simulink model "sm_dump_trailer"  (R2021b)
settings: Solver=VariableStepAuto  StartTime=0.0  StopTime=10  FixedStep=0.0001  RelTol=1e-3  AbsTol=1e-3  EnableMultiTasking=on
model workspace: external: MATLAB File sm_dump_trailer_params.m (data not in the file)
undefined symbols (not defined in the file or in its folder): base, bed, cylinder, lowerarm, sigbuilder_block, upperarm, X, Y, Z
libraries: sm_lib x65, sm_dump_trailer_lib x20, fl_lib x7, nesl_utility x4, simulink x4, sm_interface_elements_lib x1
(part 1 of 3)
CloseFcn:
  | clear simlog_sm_dump_trailer
Description:
  | Hydraulic Interface - Dump Trailer with Hydraulic Cylinder
settings Model: Creator=The MathWorks, Inc.  LastModifiedBy=The MathWorks, Inc.
settings SolverCC: AutoScaleAbsTol=off  AlgebraicLoopSolver=TrustRegion
settings DataIOCC: SaveFormat=StructureWithTime  SaveOutput=off  SignalLogging=off  DSMLogging=off  SaveTime=off  ReturnWorkspaceOutputs=off  ReturnWorkspaceOutputsName=spidata
settings DebuggingCC: SFMachineParentedDataDiag=warning  ArithmeticOperatorsInVariantConditions=warning
settings SFSimCC: SimUseLocalCustomCode=off  CustomCodeUndefinedFunction=UseInterfaceOnly
settings RTWCC: RTWUseLocalCustomCode=off
settings CodeAppCC: StateflowObjectComments=on
settings GRTTargetCC: TargetLangStandard=C89/C90 (ANSI)
settings ConfigComp: CovMetricSettings=dw  CovSaveCumulativeToWorkspaceVar=on  CovSaveSingleToWorkspaceVar=on  CovExternalEMLEnable=off
settings SimscapeCC: SimscapeNormalizeSystem=off  SimscapeLogType=all  SimscapeLogSimulationStatistics=on  SimscapeLogName=simlog_sm_dump_trailer  SimscapeLogDataHistory=10000
settings ExplorerConfigSet: InternalSimMechanicsExplorerSettings="<ExplorerConfiguration><canonicalview>default</canonicalview><AnimationSetting><BasePlaybackSpeed>1.0</BasePlaybackSpeed><PlaybackSpeedFactor>1.0</PlaybackSpeedFactor></AnimationSetting><TilePanel><TileInfo><Tiles Columns=\"1\" Count=\"1\" Rows=\"1\"><Column Left=\"2\" Weight=\"1\"/><Column Left=\"535\"/><Row Top=\"2\" Weight=\"1\"/><Row Top=\"498\"/><Tile Height=\"1\" Width=\"1\" X=\"0\" Y=\"0\"/></Tiles></TileInfo><SceneInfo><SceneViewer><BGColor><R>0.60000002384185791</R><G>0.60000002384185791</G><B>0.60000002384185791</B></BGColor><Camera><DoPerspective>off</DoPerspective><Position><X>1.5277086158018158</X><Y>0.21029843104978743</Y><Z>2.2318283328195734</Z></Position><Center><X>-0.21869209269767445</X><Y>1.956699139549277</Y><Z>0.48542762432009623</Z></Center><Up><X>-0.40824829046386307</X><Y>0.40824829046386307</Y><Z>0.81649658092772615</Z></Up><ViewLimDist>1</ViewLimDist><YLim>1.9305354565325132</YLim><XLim>2.0772085815668109</XLim></Camera></SceneViewer></SceneInfo></TilePanel><MechEditorPanel><Cameras/><GfxPanelCameraMap/><VideoCreator><PlaybackSpeedRatio>1.0</PlaybackSpeedRatio><FrameRate>30</FrameRate><VideoFormat>Motion JPEG AVI</VideoFormat><FrameSize>auto</FrameSize></VideoCreator></MechEditorPanel></ExplorerConfiguration>"

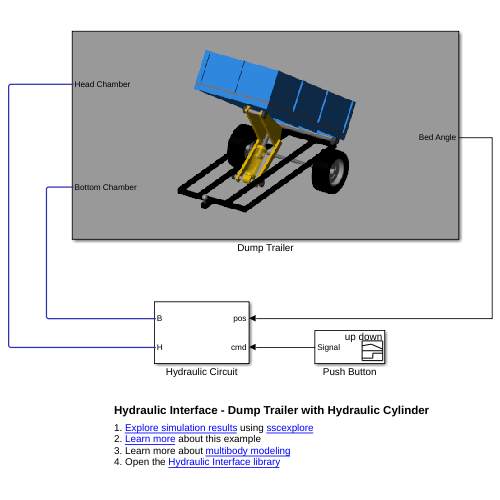
[thumbnail: Simulink's stored preview of the top-level diagram]
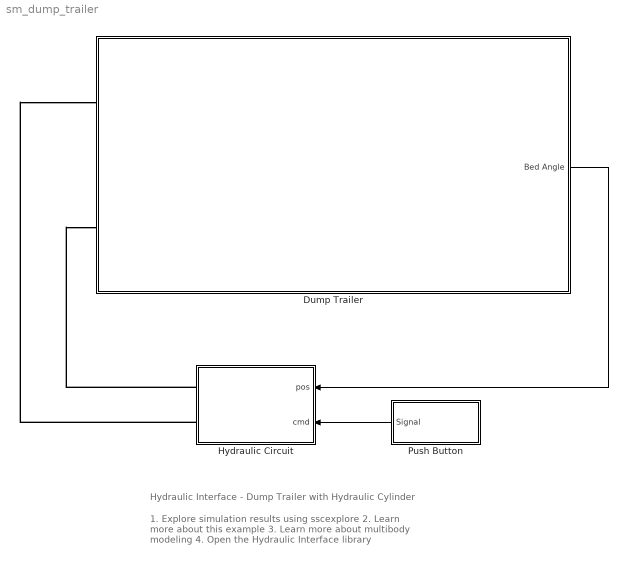
== system sm_dump_trailer ==
  note: Hydraulic Interface - Dump Trailer with Hydraulic Cylinder
  note: 1. Explore simulation results using sscexplore
      | 2. Learn more about this example
      | 3. Learn more about multibody modeling
      | 4. Open the Hydraulic Interface library
  Dump Trailer : Subsystem
      mask Display: image(fullfile(matlabroot,'toolbox','physmod','sm','smdemos','dump_trailer','images','sm_dump_trailer.png'));
  Hydraulic Circuit : Subsystem
  Push Button : Subsystem  Tag=STV Subsys  LoadFcn=sigbuilder_block('load');  StartFcn=sigbuilder_block('start');  StopFcn=sigbuilder_block('stop');  ClipboardFcn=sigbuilder_block('clipboard');  mask(Sigbuilder block){tuvar=[0:10]}
      mask help: Simulink:masks:SigbuilderBlock_MD
      mask init:
      | if ~strcmp(get_param(bdroot(gcbh),'SimulationStatus'),'stopped') tuvar = sigbuilder_block('maskInit'); end
      settings: CopyFcn=sigbuilder_block('copy');  DeleteFcn=sigbuilder_block('delete');  ModelCloseFcn=sigbuilder_block('modelClose');  PreSaveFcn=sigbuilder_block('preSave');  PauseFcn=sigbuilder_block('pause');  ContinueFcn=sigbuilder_block('continue');  NameChangeFcn=sigbuilder_block('namechange');  OpenFcn=sigbuilder_block('open',[547.5 174.75 550.5 399.75 ]);  CloseFcn=sigbuilder_block('close');
      mask Display: plot(0, 0, 100, 100,[2, 2, 32, 32, 2], [68, 8, 8, 68, 68],[32, 2], [38, 38], [32, 19, 2],[53, 60, 44], [32, 17, 17, 2],[16, 16, 31, 31]);txt = getActiveGroup(gcbh);text(2, 100, txt,'verticalAlignment', 'top');
  wires:
  Dump Trailer/1(Bed Angle) -> Hydraulic Circuit/2(pos)
  Push Button/1(Signal) -> Hydraulic Circuit/1(cmd)
  connections:
  Hydraulic Circuit/RConn2 -- Dump Trailer/LConn2
  Hydraulic Circuit/RConn1 -- Dump Trailer/LConn1

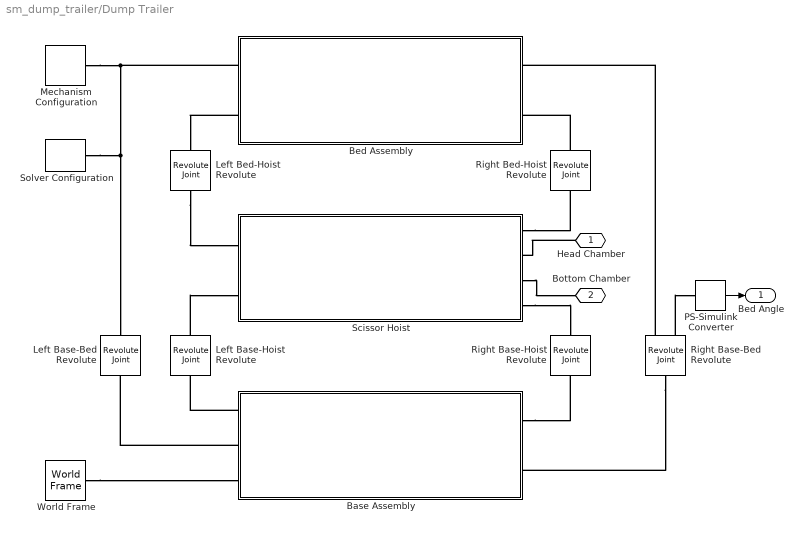
== system sm_dump_trailer/Dump Trailer ==
  Base Assembly : Subsystem
      mask Display: image(fullfile(matlabroot,'toolbox','physmod','sm','smdemos','dump_trailer','images','sm_dump_trailer_base_assembly.png'));
  Bed Assembly : Subsystem
      mask Display: image(fullfile(matlabroot,'toolbox','physmod','sm','smdemos','dump_trailer','images','sm_dump_trailer_bed_assembly.png'));
  Left Base-Bed Revolute : sm_lib/Joints/Revolute Joint  JointMode=Normal  SenseConstraintForce=off  SenseConstraintForceX=off  SenseConstraintForceY=off  SenseConstraintForceZ=off  SenseConstraintTorque=off  SenseConstraintTorqueX=off  SenseConstraintTorqueY=off  SenseConstraintTorqueZ=off  SenseTotalForce=off  SenseTotalForceX=off  SenseTotalForceY=off  SenseTotalForceZ=off  SenseTotalTorque=off  SenseTotalTorqueX=off  SenseTotalTorqueY=off  SenseTotalTorqueZ=off  CompositeWrenchDir=FollowerOnBase  CompositeWrenchFrame=BaseFrame  EquilibriumPosition=0  EquilibriumPositionUnits=deg  SpringStiffness=0  SpringStiffnessUnits=N*m/deg  DampingCoefficient=0  DampingCoefficientUnits=N*m/(deg/s)  TorqueActuationMode=NoTorque  MotionActuationMode=ComputedMotion  SensePosition=off  SenseVelocity=off  SenseAcceleration=off  SenseTorqueForce=off  SenseLowerLimitTorqueForce=off  SenseUpperLimitTorqueForce=off  LowerLimitSpecify=off  LowerLimitBound=-90  LowerLimitBoundUnits=deg  LowerLimitStiffness=1e4  LowerLimitStiffnessUnits=N*m/deg  LowerLimitDamping=10  LowerLimitDampingUnits=N*m/(deg/s)  LowerLimitTransitionRegionWidth=0.1  LowerLimitTransitionRegionWidthUnits=deg  UpperLimitSpecify=off  UpperLimitBound=90  UpperLimitBoundUnits=deg  UpperLimitStiffness=1e4  UpperLimitStiffnessUnits=N*m/deg  UpperLimitDamping=10  UpperLimitDampingUnits=N*m/(deg/s)  UpperLimitTransitionRegionWidth=0.1  UpperLimitTransitionRegionWidthUnits=deg  PositionTargetSpecify=off  PositionTargetPriority=High  PositionTargetValue=180  PositionTargetValueUnits=deg  VelocityTargetSpecify=off  VelocityTargetPriority=High  VelocityTargetValue=0  VelocityTargetValueUnits=deg/s
  Left Base-Hoist Revolute : sm_lib/Joints/Revolute Joint  JointMode=Normal  SenseConstraintForce=off  SenseConstraintForceX=off  SenseConstraintForceY=off  SenseConstraintForceZ=off  SenseConstraintTorque=off  SenseConstraintTorqueX=off  SenseConstraintTorqueY=off  SenseConstraintTorqueZ=off  SenseTotalForce=off  SenseTotalForceX=off  SenseTotalForceY=off  SenseTotalForceZ=off  SenseTotalTorque=off  SenseTotalTorqueX=off  SenseTotalTorqueY=off  SenseTotalTorqueZ=off  CompositeWrenchDir=FollowerOnBase  CompositeWrenchFrame=BaseFrame  EquilibriumPosition=0  EquilibriumPositionUnits=deg  SpringStiffness=0  SpringStiffnessUnits=N*m/deg  DampingCoefficient=0  DampingCoefficientUnits=N*m/(deg/s)  TorqueActuationMode=NoTorque  MotionActuationMode=ComputedMotion  SensePosition=off  SenseVelocity=off  SenseAcceleration=off  SenseTorqueForce=off  SenseLowerLimitTorqueForce=off  SenseUpperLimitTorqueForce=off  LowerLimitSpecify=off  LowerLimitBound=-90  LowerLimitBoundUnits=deg  LowerLimitStiffness=1e4  LowerLimitStiffnessUnits=N*m/deg  LowerLimitDamping=10  LowerLimitDampingUnits=N*m/(deg/s)  LowerLimitTransitionRegionWidth=0.1  LowerLimitTransitionRegionWidthUnits=deg  UpperLimitSpecify=off  UpperLimitBound=90  UpperLimitBoundUnits=deg  UpperLimitStiffness=1e4  UpperLimitStiffnessUnits=N*m/deg  UpperLimitDamping=10  UpperLimitDampingUnits=N*m/(deg/s)  UpperLimitTransitionRegionWidth=0.1  UpperLimitTransitionRegionWidthUnits=deg  PositionTargetSpecify=on  PositionTargetPriority=Low  PositionTargetValue=185  PositionTargetValueUnits=deg  VelocityTargetSpecify=off  VelocityTargetPriority=High  VelocityTargetValue=0  VelocityTargetValueUnits=deg/s
  Left Bed-Hoist Revolute : sm_lib/Joints/Revolute Joint  JointMode=Normal  SenseConstraintForce=off  SenseConstraintForceX=off  SenseConstraintForceY=off  SenseConstraintForceZ=off  SenseConstraintTorque=off  SenseConstraintTorqueX=off  SenseConstraintTorqueY=off  SenseConstraintTorqueZ=off  SenseTotalForce=off  SenseTotalForceX=off  SenseTotalForceY=off  SenseTotalForceZ=off  SenseTotalTorque=off  SenseTotalTorqueX=off  SenseTotalTorqueY=off  SenseTotalTorqueZ=off  CompositeWrenchDir=FollowerOnBase  CompositeWrenchFrame=BaseFrame  EquilibriumPosition=0  EquilibriumPositionUnits=deg  SpringStiffness=0  SpringStiffnessUnits=N*m/deg  DampingCoefficient=0  DampingCoefficientUnits=N*m/(deg/s)  TorqueActuationMode=NoTorque  MotionActuationMode=ComputedMotion  SensePosition=off  SenseVelocity=off  SenseAcceleration=off  SenseTorqueForce=off  SenseLowerLimitTorqueForce=off  SenseUpperLimitTorqueForce=off  LowerLimitSpecify=off  LowerLimitBound=-90  LowerLimitBoundUnits=deg  LowerLimitStiffness=1e4  LowerLimitStiffnessUnits=N*m/deg  LowerLimitDamping=10  LowerLimitDampingUnits=N*m/(deg/s)  LowerLimitTransitionRegionWidth=0.1  LowerLimitTransitionRegionWidthUnits=deg  UpperLimitSpecify=off  UpperLimitBound=90  UpperLimitBoundUnits=deg  UpperLimitStiffness=1e4  UpperLimitStiffnessUnits=N*m/deg  UpperLimitDamping=10  UpperLimitDampingUnits=N*m/(deg/s)  UpperLimitTransitionRegionWidth=0.1  UpperLimitTransitionRegionWidthUnits=deg  PositionTargetSpecify=off  PositionTargetPriority=High  PositionTargetValue=0  PositionTargetValueUnits=deg  VelocityTargetSpecify=off  VelocityTargetPriority=High  VelocityTargetValue=0  VelocityTargetValueUnits=deg/s
  Mechanism Configuration : sm_lib/Utilities/Mechanism Configuration  UniformGravity=Constant  GravityVector=[0 0 -9.80665]  GravityUnits=m/s^2  LinearizationDelta=0.001  JointModeTransitionNonlinearIterations=2
  PS-Simulink Converter : nesl_utility/PS-Simulink Converter  PhysicalDomain=network_engine_domain  SubClassName=ps_output  LeftPortType=input  RightPortType=output  PseudoPeriodic=off  Frequencies=[]  Unit=deg  AffineConversion=off
      settings: SourceProductBaseCode=PW,SS
  Right Base-Bed Revolute : sm_lib/Joints/Revolute Joint  JointMode=Normal  SenseConstraintForce=off  SenseConstraintForceX=off  SenseConstraintForceY=off  SenseConstraintForceZ=off  SenseConstraintTorque=off  SenseConstraintTorqueX=off  SenseConstraintTorqueY=off  SenseConstraintTorqueZ=off  SenseTotalForce=off  SenseTotalForceX=off  SenseTotalForceY=off  SenseTotalForceZ=off  SenseTotalTorque=off  SenseTotalTorqueX=off  SenseTotalTorqueY=off  SenseTotalTorqueZ=off  CompositeWrenchDir=FollowerOnBase  CompositeWrenchFrame=BaseFrame  EquilibriumPosition=0  EquilibriumPositionUnits=deg  SpringStiffness=0  SpringStiffnessUnits=N*m/deg  DampingCoefficient=0  DampingCoefficientUnits=N*m/(deg/s)  TorqueActuationMode=NoTorque  MotionActuationMode=ComputedMotion  SensePosition=on  SenseVelocity=off  SenseAcceleration=off  SenseTorqueForce=off  SenseLowerLimitTorqueForce=off  SenseUpperLimitTorqueForce=off  LowerLimitSpecify=off  LowerLimitBound=-90  LowerLimitBoundUnits=deg  LowerLimitStiffness=1e4  LowerLimitStiffnessUnits=N*m/deg  LowerLimitDamping=10  LowerLimitDampingUnits=N*m/(deg/s)  LowerLimitTransitionRegionWidth=0.1  LowerLimitTransitionRegionWidthUnits=deg  UpperLimitSpecify=off  UpperLimitBound=90  UpperLimitBoundUnits=deg  UpperLimitStiffness=1e4  UpperLimitStiffnessUnits=N*m/deg  UpperLimitDamping=10  UpperLimitDampingUnits=N*m/(deg/s)  UpperLimitTransitionRegionWidth=0.1  UpperLimitTransitionRegionWidthUnits=deg  PositionTargetSpecify=on  PositionTargetPriority=High  PositionTargetValue=0  PositionTargetValueUnits=deg  VelocityTargetSpecify=off  VelocityTargetPriority=High  VelocityTargetValue=0  VelocityTargetValueUnits=deg/s
  Right Base-Hoist Revolute : sm_lib/Joints/Revolute Joint  JointMode=Normal  SenseConstraintForce=off  SenseConstraintForceX=off  SenseConstraintForceY=off  SenseConstraintForceZ=off  SenseConstraintTorque=off  SenseConstraintTorqueX=off  SenseConstraintTorqueY=off  SenseConstraintTorqueZ=off  SenseTotalForce=off  SenseTotalForceX=off  SenseTotalForceY=off  SenseTotalForceZ=off  SenseTotalTorque=off  SenseTotalTorqueX=off  SenseTotalTorqueY=off  SenseTotalTorqueZ=off  CompositeWrenchDir=FollowerOnBase  CompositeWrenchFrame=BaseFrame  EquilibriumPosition=0  EquilibriumPositionUnits=deg  SpringStiffness=0  SpringStiffnessUnits=N*m/deg  DampingCoefficient=0  DampingCoefficientUnits=N*m/(deg/s)  TorqueActuationMode=NoTorque  MotionActuationMode=ComputedMotion  SensePosition=off  SenseVelocity=off  SenseAcceleration=off  SenseTorqueForce=off  SenseLowerLimitTorqueForce=off  SenseUpperLimitTorqueForce=off  LowerLimitSpecify=off  LowerLimitBound=-90  LowerLimitBoundUnits=deg  LowerLimitStiffness=1e4  LowerLimitStiffnessUnits=N*m/deg  LowerLimitDamping=10  LowerLimitDampingUnits=N*m/(deg/s)  LowerLimitTransitionRegionWidth=0.1  LowerLimitTransitionRegionWidthUnits=deg  UpperLimitSpecify=off  UpperLimitBound=90  UpperLimitBoundUnits=deg  UpperLimitStiffness=1e4  UpperLimitStiffnessUnits=N*m/deg  UpperLimitDamping=10  UpperLimitDampingUnits=N*m/(deg/s)  UpperLimitTransitionRegionWidth=0.1  UpperLimitTransitionRegionWidthUnits=deg  PositionTargetSpecify=off  PositionTargetPriority=High  PositionTargetValue=0  PositionTargetValueUnits=deg  VelocityTargetSpecify=off  VelocityTargetPriority=High  VelocityTargetValue=0  VelocityTargetValueUnits=deg/s
  Right Bed-Hoist Revolute : sm_lib/Joints/Revolute Joint  JointMode=Normal  SenseConstraintForce=off  SenseConstraintForceX=off  SenseConstraintForceY=off  SenseConstraintForceZ=off  SenseConstraintTorque=off  SenseConstraintTorqueX=off  SenseConstraintTorqueY=off  SenseConstraintTorqueZ=off  SenseTotalForce=off  SenseTotalForceX=off  SenseTotalForceY=off  SenseTotalForceZ=off  SenseTotalTorque=off  SenseTotalTorqueX=off  SenseTotalTorqueY=off  SenseTotalTorqueZ=off  CompositeWrenchDir=FollowerOnBase  CompositeWrenchFrame=BaseFrame  EquilibriumPosition=0  EquilibriumPositionUnits=deg  SpringStiffness=0  SpringStiffnessUnits=N*m/deg  DampingCoefficient=0  DampingCoefficientUnits=N*m/(deg/s)  TorqueActuationMode=NoTorque  MotionActuationMode=ComputedMotion  SensePosition=off  SenseVelocity=off  SenseAcceleration=off  SenseTorqueForce=off  SenseLowerLimitTorqueForce=off  SenseUpperLimitTorqueForce=off  LowerLimitSpecify=off  LowerLimitBound=-90  LowerLimitBoundUnits=deg  LowerLimitStiffness=1e4  LowerLimitStiffnessUnits=N*m/deg  LowerLimitDamping=10  LowerLimitDampingUnits=N*m/(deg/s)  LowerLimitTransitionRegionWidth=0.1  LowerLimitTransitionRegionWidthUnits=deg  UpperLimitSpecify=off  UpperLimitBound=90  UpperLimitBoundUnits=deg  UpperLimitStiffness=1e4  UpperLimitStiffnessUnits=N*m/deg  UpperLimitDamping=10  UpperLimitDampingUnits=N*m/(deg/s)  UpperLimitTransitionRegionWidth=0.1  UpperLimitTransitionRegionWidthUnits=deg  PositionTargetSpecify=off  PositionTargetPriority=High  PositionTargetValue=0  PositionTargetValueUnits=deg  VelocityTargetSpecify=off  VelocityTargetPriority=High  VelocityTargetValue=0  VelocityTargetValueUnits=deg/s
  Scissor Hoist : Subsystem
      mask Display: image(fullfile(matlabroot,'toolbox','physmod','sm','smdemos','dump_trailer','images','sm_dump_trailer_scissor_hoist.png'));
  Solver Configuration : nesl_utility/Solver Configuration  PhysicalDomain=network_engine_domain  SubClassName=solver  LeftPortType=input  RightPortType=generic  Tones=[]  Harmonics=[]  SimulateNoise=off  Profile=off  UseLocalSampling=off  EnableSwitchedLinearOptims=on  FrequencyDomain=off  UseCCode=off  RelTol=0.001  AbsTol=1e-06  MinStep=1e-09  ToWorkspace=off  RevertToSquareIcSolve=off  NumHomotopyIterations=100  PhasorMode=off  PhasorModeNumHarmonics=1  DoDC=off  ResidualTolerance=1e-09  UseLocalSolver=off  LocalSolverChoice=NE_BACKWARD_EULER_ADVANCER  LocalSolverSampleTime=0.001  DoFixedCost=off  MaxNonlinIter=3  MaxModeIter=2  ComputeImpulses=off  ImpulseIterations=2  LinearAlgebra=Sparse  EquationFormulation=NE_TIME_EF  DelaysMemoryBudget=1024  AutomaticFiltering=on  FilteringTimeConstant=0.001  PartitionStorageMethod=AS_NEEDED  PartitionMemoryBudget=1024  PartitionMethod=FAST
      settings: SourceProductBaseCode=PW,SS
  World Frame : sm_lib/Frames and Transforms/World Frame
  Head Chamber : PMIOPort  Side=Left
  Bottom Chamber : PMIOPort  Port=2  Side=Left
  Bed Angle : Outport  VectorParamsAs1DForOutWhenUnconnected=off
  wires:
  PS-Simulink Converter/1 -> Bed Angle/1
  connections:
  Scissor Hoist/RConn3 -- Bottom Chamber/RConn1
  Head Chamber/RConn1 -- Scissor Hoist/RConn2
  Base Assembly/RConn1 -- Right Base-Hoist Revolute/LConn1
  Scissor Hoist/RConn4 -- Right Base-Hoist Revolute/RConn1
  Left Base-Hoist Revolute/RConn1 -- Scissor Hoist/LConn2
  Base Assembly/LConn1 -- Left Base-Hoist Revolute/LConn1
  Left Bed-Hoist Revolute/RConn1 -- Scissor Hoist/LConn1
  Scissor Hoist/RConn1 -- Right Bed-Hoist Revolute/RConn1
  Base Assembly/LConn2 -- Left Base-Bed Revolute/LConn1
  Right Base-Bed Revolute/LConn1 -- Base Assembly/RConn2
  Bed Assembly/LConn1 -- Mechanism Configuration/RConn1 -- Solver Configuration/RConn1 -- Left Base-Bed Revolute/RConn1
  Right Base-Bed Revolute/RConn1 -- Bed Assembly/RConn1
  World Frame/RConn1 -- Base Assembly/LConn3
  Right Bed-Hoist Revolute/LConn1 -- Bed Assembly/RConn2
  Bed Assembly/LConn2 -- Left Bed-Hoist Revolute/LConn1
  Right Base-Bed Revolute/RConn2 -- PS-Simulink Converter/LConn1

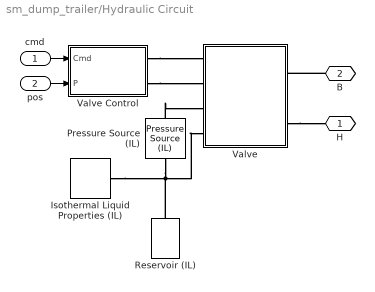
== system sm_dump_trailer/Hydraulic Circuit ==
  cmd : Inport
  pos : Inport  Port=2
  Isothermal Liquid Properties (IL) : fl_lib/Isothermal Liquid/Utilities/Isothermal Liquid Properties (IL)  rho_L_atm=850 kg/m^3  bulk_modulus_model=foundation.enum.bulk_modulus_model.const  beta_gain=6  beta_L_atm=8e+08 Pa  nu_atm=1.8e-05 m^2/s  p_atm=0.101325 MPa  p_min=0.1 Pa  air_fraction=0.005  polytropic_index=1.0  rho_g_atm=1.225 kg/m^3  air_dissolution_model=simscape.enum.onoff.off  p_crit=3 MPa
      settings: SourceProductBaseCode=SS
  Pressure Source (IL) : fl_lib/Isothermal Liquid/Sources/Pressure Source (IL)  source_type=foundation.enum.constant_controlled.constant  pressure_differential=4e7 Pa
      settings: SourceProductBaseCode=SS  InternalSimscapePortConfiguration="{\"Bottom\":[],\"Left\":[{\"id\":\"A\",\"label\":\"A\",\"type\":\"foundation.isothermal_liquid.isothermal_liquid\"}],\"Right\":[{\"id\":\"B\",\"label\":\"B\",\"type\":\"foundation.isothermal_liquid.isothermal_liquid\"}],\"Top\":[]}"
  Reservoir (IL) : fl_lib/Isothermal Liquid/Elements/Reservoir (IL)  reservoir_type=foundation.enum.constant_controlled.constant  pressure_spec=foundation.enum.pressure_spec.atmospheric  reservoir_pressure=0.101325 MPa
      settings: SourceProductBaseCode=SS
  Valve : Subsystem
  Valve Control : Subsystem
  H : PMIOPort  Side=Right
  B : PMIOPort  Port=2  Side=Right
  wires:
  cmd/1 -> Valve Control/1(Cmd)
  pos/1 -> Valve Control/2(P)
  connections:
  Valve/LConn4 -- Reservoir (IL)/LConn1 -- Isothermal Liquid Properties (IL)/RConn1 -- Pressure Source (IL)/LConn1
  Valve Control/RConn1 -- Valve/LConn1
  Valve Control/RConn2 -- Valve/LConn2
  B/RConn1 -- Valve/RConn1
  Valve/RConn2 -- H/RConn1
  Pressure Source (IL)/RConn1 -- Valve/LConn3

== system sm_dump_trailer/Push Button ==
  Demux : Demux  Tag=STV Demux  Outputs=1
      settings: DisplayOption=none
  FromWs : FromWorkspace  Tag=STV FromWs  VariableName=tuvar
      SigBuilderData=|
      | common.afterFinalStr = 'Extrapolate'
      | common.sampleTime = 0
      | dataSet.timeRange = [0 10]
      | dataSet.name = 'up down'
      | sbobj.Groups.Name = 'up down'
      | sbobj.Groups.Signals.Name = 'Signal'
      | sbobj.Groups.Signals.XData = [0 1 1 2.98 2.98 6 6 9 9 10]
      | sbobj.Groups.Signals.YData = [0 0 1 1 0 0 -1 -1 0 -0.001]
  Signal : Outport  Tag=STV Outport  VectorParamsAs1DForOutWhenUnconnected=off
  wires:
  Demux/1 -> Signal/1
  FromWs/1 -> Demux/1

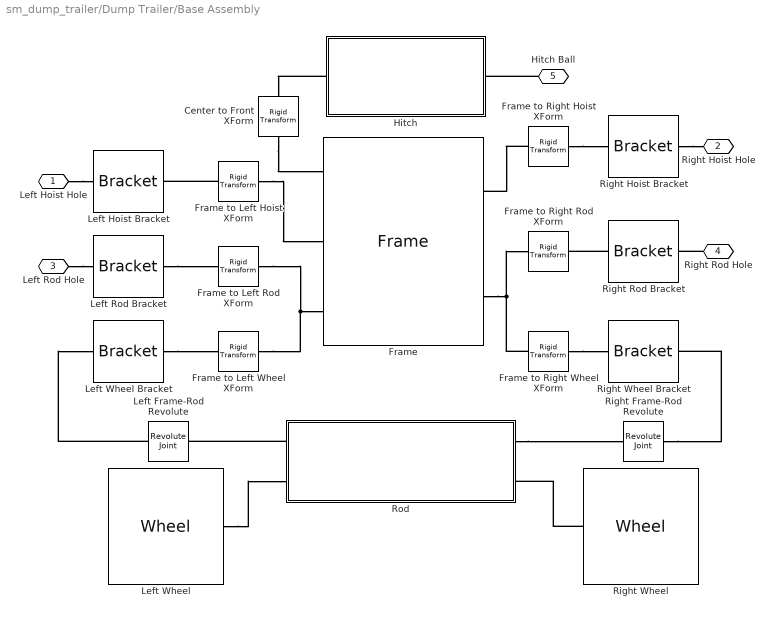
== system sm_dump_trailer/Dump Trailer/Base Assembly ==
  Center to Front XForm : sm_lib/Frames and Transforms/Rigid Transform  TranslationMethod=StandardAxis  TranslationStandardOffset=base.frame.length/2  TranslationLengthUnit=m  TranslationStandardAxis=-Y  TranslationCartesianOffset=[0 0 0]  TranslationROffset=0  TranslationROffsetUnits=m  TranslationZOffset=0  TranslationZOffsetUnits=m  TranslationThetaOffset=0  TranslationThetaOffsetUnits=deg  RotationMethod=None  RotationAngleUnits=deg  RotationStandardAxis=-Z  RotationAngle=90  RotationArbitraryAxis=[0 0 1]  FollAlignAxisA=+X  BaseAlignAxisA=+Y  FollAlignAxisB=+Y  BaseAlignAxisB=+Z  RotationSequenceAxes=FollowerAxes  RotationSequence=XYX  RotationSequenceAngles=[0 0 0]  RotationSequenceAnglesUnits=deg  RotationMatrix=[1 0 0; 0 1 0; 0 0 1]
  Frame : sm_dump_trailer_lib/Frame  W=base.frame.width  L=base.frame.length  H=base.frame.height  T=base.frame.thickness  d_innerbeams=base.frame.innerbeamdistance  rho=base.frame.density  color=base.frame.color
      settings: SourceProductBaseCode=MS
  Frame to Left Hoist XForm : sm_lib/Frames and Transforms/Rigid Transform  TranslationMethod=Cartesian  TranslationStandardOffset=0  TranslationLengthUnit=m  TranslationStandardAxis=+Z  TranslationCartesianOffset=base.hoistbracket.offset  TranslationROffset=0  TranslationROffsetUnits=m  TranslationZOffset=0  TranslationZOffsetUnits=m  TranslationThetaOffset=0  TranslationThetaOffsetUnits=deg  RotationMethod=StandardAxis  RotationAngleUnits=deg  RotationStandardAxis=+Y  RotationAngle=180  RotationArbitraryAxis=[0 0 1]  FollAlignAxisA=+X  BaseAlignAxisA=+Y  FollAlignAxisB=+Y  BaseAlignAxisB=+Z  RotationSequenceAxes=FollowerAxes  RotationSequence=XYX  RotationSequenceAngles=[0 0 0]  RotationSequenceAnglesUnits=deg  RotationMatrix=[1 0 0; 0 1 0; 0 0 1]
  Frame to Left Rod XForm : sm_lib/Frames and Transforms/Rigid Transform  TranslationMethod=Cartesian  TranslationStandardOffset=0  TranslationLengthUnit=m  TranslationStandardAxis=+Z  TranslationCartesianOffset=base.rodbracket.offset  TranslationROffset=0  TranslationROffsetUnits=m  TranslationZOffset=0  TranslationZOffsetUnits=m  TranslationThetaOffset=0  TranslationThetaOffsetUnits=deg  RotationMethod=None  RotationAngleUnits=deg  RotationStandardAxis=+Y  RotationAngle=180  RotationArbitraryAxis=[0 0 1]  FollAlignAxisA=+X  BaseAlignAxisA=+Y  FollAlignAxisB=+Y  BaseAlignAxisB=+Z  RotationSequenceAxes=FollowerAxes  RotationSequence=XYX  RotationSequenceAngles=[0 0 0]  RotationSequenceAnglesUnits=deg  RotationMatrix=[1 0 0; 0 1 0; 0 0 1]
  Frame to Left Wheel XForm : sm_lib/Frames and Transforms/Rigid Transform  TranslationMethod=Cartesian  TranslationStandardOffset=0  TranslationLengthUnit=m  TranslationStandardAxis=+Z  TranslationCartesianOffset=base.wheelbracket.offset  TranslationROffset=0  TranslationROffsetUnits=m  TranslationZOffset=0  TranslationZOffsetUnits=m  TranslationThetaOffset=0  TranslationThetaOffsetUnits=deg  RotationMethod=StandardAxis  RotationAngleUnits=deg  RotationStandardAxis=+Y  RotationAngle=180  RotationArbitraryAxis=[0 0 1]  FollAlignAxisA=+X  BaseAlignAxisA=+Y  FollAlignAxisB=+Y  BaseAlignAxisB=+Z  RotationSequenceAxes=FollowerAxes  RotationSequence=XYX  RotationSequenceAngles=[0 0 0]  RotationSequenceAnglesUnits=deg  RotationMatrix=[1 0 0; 0 1 0; 0 0 1]
  Frame to Right Hoist XForm : sm_lib/Frames and Transforms/Rigid Transform  TranslationMethod=Cartesian  TranslationStandardOffset=0  TranslationLengthUnit=m  TranslationStandardAxis=+Z  TranslationCartesianOffset=base.hoistbracket.offset  TranslationROffset=0  TranslationROffsetUnits=m  TranslationZOffset=0  TranslationZOffsetUnits=m  TranslationThetaOffset=0  TranslationThetaOffsetUnits=deg  RotationMethod=StandardAxis  RotationAngleUnits=deg  RotationStandardAxis=+Y  RotationAngle=180  RotationArbitraryAxis=[0 0 1]  FollAlignAxisA=+X  BaseAlignAxisA=+Y  FollAlignAxisB=+Y  BaseAlignAxisB=+Z  RotationSequenceAxes=FollowerAxes  RotationSequence=XYX  RotationSequenceAngles=[0 0 0]  RotationSequenceAnglesUnits=deg  RotationMatrix=[1 0 0; 0 1 0; 0 0 1]
  Frame to Right Rod XForm : sm_lib/Frames and Transforms/Rigid Transform  TranslationMethod=Cartesian  TranslationStandardOffset=0  TranslationLengthUnit=m  TranslationStandardAxis=+Z  TranslationCartesianOffset=base.rodbracket.offset  TranslationROffset=0  TranslationROffsetUnits=m  TranslationZOffset=0  TranslationZOffsetUnits=m  TranslationThetaOffset=0  TranslationThetaOffsetUnits=deg  RotationMethod=StandardAxis  RotationAngleUnits=deg  RotationStandardAxis=+Z  RotationAngle=180  RotationArbitraryAxis=[0 0 1]  FollAlignAxisA=+X  BaseAlignAxisA=+Y  FollAlignAxisB=+Y  BaseAlignAxisB=+Z  RotationSequenceAxes=FollowerAxes  RotationSequence=XYX  RotationSequenceAngles=[0 0 0]  RotationSequenceAnglesUnits=deg  RotationMatrix=[1 0 0; 0 1 0; 0 0 1]
  Frame to Right Wheel XForm : sm_lib/Frames and Transforms/Rigid Transform  TranslationMethod=Cartesian  TranslationStandardOffset=0  TranslationLengthUnit=m  TranslationStandardAxis=+Z  TranslationCartesianOffset=base.wheelbracket.offset  TranslationROffset=0  TranslationROffsetUnits=m  TranslationZOffset=0  TranslationZOffsetUnits=m  TranslationThetaOffset=0  TranslationThetaOffsetUnits=deg  RotationMethod=StandardAxis  RotationAngleUnits=deg  RotationStandardAxis=+Y  RotationAngle=180  RotationArbitraryAxis=[0 0 1]  FollAlignAxisA=+X  BaseAlignAxisA=+Y  FollAlignAxisB=+Y  BaseAlignAxisB=+Z  RotationSequenceAxes=FollowerAxes  RotationSequence=XYX  RotationSequenceAngles=[0 0 0]  RotationSequenceAnglesUnits=deg  RotationMatrix=[1 0 0; 0 1 0; 0 0 1]
  Hitch : Subsystem  mask{L_bar=base.hitch.bar.length, W_bar=base.hitch.bar.width, H_bar=base.hitch.bar.height, rho_bar=base.hitch.bar.density, color_bar=base.hitch.bar.color, r_cyl=base.hitch.cylinder.radius, L_cyl=base.hitch.cylinder.length, d_cyl_offset=base.hitch.cylinder.offset, rho_cyl=base.hitch.cylinder.density, color_cyl=base.hitch.cylinder.color, r_ball=base.hitch.ball.radius, rho_ball=base.hitch.ball.density, color_ball=base.hitch.ball.color}
      mask prompts: L_bar "Length (m)"; W_bar "Width (m)"; H_bar "Height (m)"; rho_bar "Density (kg/m^3)"; color_bar "Color [R G B]"; r_cyl "Radius (m)"; L_cyl "Length (m)"; d_cyl_offset "Offset from frame (m)"; rho_cyl "Density (kg/m^3)"; color_cyl "Color [R G B]"; r_ball "Radius (m)"; rho_ball "Density (kg/m^3)"; color_ball "Color [R G B]"
      mask DialogControl Container4 Prompt: Bar
      mask DialogControl Container5 Prompt: Cylinder
      mask DialogControl Container6 Prompt: Ball
      mask Display: image(fullfile(matlabroot,'toolbox','physmod','sm','smdemos','dump_trailer','images','sm_dump_trailer_hitch.png'));
  Left Frame-Rod Revolute : sm_lib/Joints/Revolute Joint  JointMode=Normal  SenseConstraintForce=off  SenseConstraintForceX=off  SenseConstraintForceY=off  SenseConstraintForceZ=off  SenseConstraintTorque=off  SenseConstraintTorqueX=off  SenseConstraintTorqueY=off  SenseConstraintTorqueZ=off  SenseTotalForce=off  SenseTotalForceX=off  SenseTotalForceY=off  SenseTotalForceZ=off  SenseTotalTorque=off  SenseTotalTorqueX=off  SenseTotalTorqueY=off  SenseTotalTorqueZ=off  CompositeWrenchDir=FollowerOnBase  CompositeWrenchFrame=BaseFrame  EquilibriumPosition=0  EquilibriumPositionUnits=deg  SpringStiffness=0  SpringStiffnessUnits=N*m/deg  DampingCoefficient=0  DampingCoefficientUnits=N*m/(deg/s)  TorqueActuationMode=NoTorque  MotionActuationMode=ComputedMotion  SensePosition=off  SenseVelocity=off  SenseAcceleration=off  SenseTorqueForce=off  SenseLowerLimitTorqueForce=off  SenseUpperLimitTorqueForce=off  LowerLimitSpecify=off  LowerLimitBound=-90  LowerLimitBoundUnits=deg  LowerLimitStiffness=1e4  LowerLimitStiffnessUnits=N*m/deg  LowerLimitDamping=10  LowerLimitDampingUnits=N*m/(deg/s)  LowerLimitTransitionRegionWidth=0.1  LowerLimitTransitionRegionWidthUnits=deg  UpperLimitSpecify=off  UpperLimitBound=90  UpperLimitBoundUnits=deg  UpperLimitStiffness=1e4  UpperLimitStiffnessUnits=N*m/deg  UpperLimitDamping=10  UpperLimitDampingUnits=N*m/(deg/s)  UpperLimitTransitionRegionWidth=0.1  UpperLimitTransitionRegionWidthUnits=deg  PositionTargetSpecify=off  PositionTargetPriority=High  PositionTargetValue=0  PositionTargetValueUnits=deg  VelocityTargetSpecify=off  VelocityTargetPriority=High  VelocityTargetValue=0  VelocityTargetValueUnits=deg/s
  Left Hoist Bracket : sm_dump_trailer_lib/Bracket  Hbracket=base.hoistbracket.height  Wbracket=base.hoistbracket.width  Tbracket=base.hoistbracket.thickness  Hhole=base.hoistbracket.holeheight  Rhole=base.hoistbracket.holeradius  rho=base.hoistbracket.density  bracketColor=base.hoistbracket.color
      settings: SourceProductBaseCode=MS
  Left Rod Bracket : sm_dump_trailer_lib/Bracket  Hbracket=base.rodbracket.height  Wbracket=base.rodbracket.width  Tbracket=base.rodbracket.thickness  Hhole=base.rodbracket.holeheight  Rhole=base.rodbracket.holeradius  rho=base.rodbracket.density  bracketColor=base.rodbracket.color
      settings: SourceProductBaseCode=MS
  Left Wheel : sm_dump_trailer_lib/Wheel  r_i=base.wheel.tire.innerradius  r_o=base.wheel.tire.outerradius  w=base.wheel.tire.width  r_c=base.wheel.tire.chamferradius  rho_tire=base.wheel.tire.density  color_tire=base.wheel.tire.color  rho_hub=base.wheel.hub.density  color_hub=base.wheel.hub.color
      settings: SourceProductBaseCode=MS
  Left Wheel Bracket : sm_dump_trailer_lib/Bracket  Hbracket=base.wheelbracket.height  Wbracket=base.wheelbracket.width  Tbracket=base.wheelbracket.thickness  Hhole=base.wheelbracket.holeheight  Rhole=base.wheelbracket.holeradius  rho=base.wheelbracket.density  bracketColor=base.wheelbracket.color
      settings: SourceProductBaseCode=MS
  Right Frame-Rod Revolute : sm_lib/Joints/Revolute Joint  JointMode=Normal  SenseConstraintForce=off  SenseConstraintForceX=off  SenseConstraintForceY=off  SenseConstraintForceZ=off  SenseConstraintTorque=off  SenseConstraintTorqueX=off  SenseConstraintTorqueY=off  SenseConstraintTorqueZ=off  SenseTotalForce=off  SenseTotalForceX=off  SenseTotalForceY=off  SenseTotalForceZ=off  SenseTotalTorque=off  SenseTotalTorqueX=off  SenseTotalTorqueY=off  SenseTotalTorqueZ=off  CompositeWrenchDir=FollowerOnBase  CompositeWrenchFrame=BaseFrame  EquilibriumPosition=0  EquilibriumPositionUnits=deg  SpringStiffness=0  SpringStiffnessUnits=N*m/deg  DampingCoefficient=0  DampingCoefficientUnits=N*m/(deg/s)  TorqueActuationMode=NoTorque  MotionActuationMode=ComputedMotion  SensePosition=off  SenseVelocity=off  SenseAcceleration=off  SenseTorqueForce=off  SenseLowerLimitTorqueForce=off  SenseUpperLimitTorqueForce=off  LowerLimitSpecify=off  LowerLimitBound=-90  LowerLimitBoundUnits=deg  LowerLimitStiffness=1e4  LowerLimitStiffnessUnits=N*m/deg  LowerLimitDamping=10  LowerLimitDampingUnits=N*m/(deg/s)  LowerLimitTransitionRegionWidth=0.1  LowerLimitTransitionRegionWidthUnits=deg  UpperLimitSpecify=off  UpperLimitBound=90  UpperLimitBoundUnits=deg  UpperLimitStiffness=1e4  UpperLimitStiffnessUnits=N*m/deg  UpperLimitDamping=10  UpperLimitDampingUnits=N*m/(deg/s)  UpperLimitTransitionRegionWidth=0.1  UpperLimitTransitionRegionWidthUnits=deg  PositionTargetSpecify=off  PositionTargetPriority=High  PositionTargetValue=0  PositionTargetValueUnits=deg  VelocityTargetSpecify=off  VelocityTargetPriority=High  VelocityTargetValue=0  VelocityTargetValueUnits=deg/s
  Right Hoist Bracket : sm_dump_trailer_lib/Bracket  Hbracket=base.hoistbracket.height  Wbracket=base.hoistbracket.width  Tbracket=base.hoistbracket.thickness  Hhole=base.hoistbracket.holeheight  Rhole=base.hoistbracket.holeradius  rho=base.hoistbracket.density  bracketColor=base.hoistbracket.color
      settings: SourceProductBaseCode=MS
  Right Rod Bracket : sm_dump_trailer_lib/Bracket  Hbracket=base.rodbracket.height  Wbracket=base.rodbracket.width  Tbracket=base.rodbracket.thickness  Hhole=base.rodbracket.holeheight  Rhole=base.rodbracket.holeradius  rho=base.rodbracket.density  bracketColor=base.rodbracket.color
      settings: SourceProductBaseCode=MS
  Right Wheel : sm_dump_trailer_lib/Wheel  r_i=base.wheel.tire.innerradius  r_o=base.wheel.tire.outerradius  w=base.wheel.tire.width  r_c=base.wheel.tire.chamferradius  rho_tire=base.wheel.tire.density  color_tire=base.wheel.tire.color  rho_hub=base.wheel.hub.density  color_hub=base.wheel.hub.color
      settings: SourceProductBaseCode=MS
  Right Wheel Bracket : sm_dump_trailer_lib/Bracket  Hbracket=base.wheelbracket.height  Wbracket=base.wheelbracket.width  Tbracket=base.wheelbracket.thickness  Hhole=base.wheelbracket.holeheight  Rhole=base.wheelbracket.holeradius  rho=base.wheelbracket.density  bracketColor=base.wheelbracket.color
      settings: SourceProductBaseCode=MS
  Rod : Subsystem  mask{L=base.rod.length, r=base.rod.radius, d_rev=base.rod.d_rev, d_wheel=base.rod.d_wheel, rho=base.rod.density, color=base.rod.color}
      mask prompts: L "Length (m)"; r "Radius (m)"; d_rev "Distance from center to revolute joints (m)"; d_wheel "Distance from center to wheels (m)"; rho "Density (kg/m^3)"; color "Color [R G B]"
      mask Display: image(fullfile(matlabroot,'toolbox','physmod','sm','smdemos','dump_trailer','images','sm_dump_trailer_rod.png'));
  Left Hoist Hole : PMIOPort  Side=Left
  Right Hoist Hole : PMIOPort  Port=2  Side=Right
  Left Rod Hole : PMIOPort  Port=3  Side=Left
  Right Rod Hole : PMIOPort  Port=4  Side=Right
  Hitch Ball : PMIOPort  Port=5  Side=Left
  connections:
  Left Hoist Hole/RConn1 -- Left Hoist Bracket/RConn1
  Frame to Right Hoist XForm/LConn1 -- Frame/RConn1
  Right Hoist Bracket/RConn1 -- Right Hoist Hole/RConn1
  Frame to Right Hoist XForm/RConn1 -- Right Hoist Bracket/LConn1
  Frame to Left Hoist XForm/RConn1 -- Left Hoist Bracket/LConn1
  Left Rod Bracket/LConn1 -- Frame to Left Rod XForm/RConn1
  Frame to Right Wheel XForm/LConn1 -- Frame to Right Rod XForm/LConn1 -- Frame/RConn2
  Right Rod Bracket/LConn1 -- Frame to Right Rod XForm/RConn1
  Frame to Left Rod XForm/LConn1 -- Frame/LConn3 -- Frame to Left Wheel XForm/LConn1
  Frame to Left Hoist XForm/LConn1 -- Frame/LConn2
  Center to Front XForm/LConn1 -- Frame/LConn1
  Right Rod Hole/RConn1 -- Right Rod Bracket/RConn1
  Left Rod Hole/RConn1 -- Left Rod Bracket/RConn1
  Left Wheel Bracket/LConn1 -- Frame to Left Wheel XForm/RConn1
  Frame to Right Wheel XForm/RConn1 -- Right Wheel Bracket/LConn1
  Left Frame-Rod Revolute/RConn1 -- Left Wheel Bracket/RConn1
  Right Frame-Rod Revolute/RConn1 -- Right Wheel Bracket/RConn1
  Right Wheel/LConn1 -- Rod/RConn2
  Left Wheel/LConn1 -- Rod/LConn2
  Rod/LConn1 -- Left Frame-Rod Revolute/LConn1
  Rod/RConn1 -- Right Frame-Rod Revolute/LConn1
  Hitch/LConn1 -- Center to Front XForm/RConn1
  Hitch Ball/RConn1 -- Hitch/RConn1

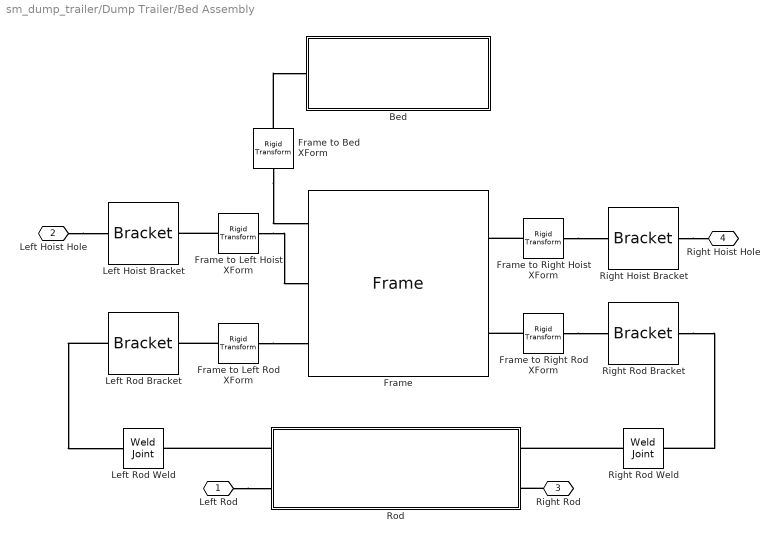
== system sm_dump_trailer/Dump Trailer/Bed Assembly ==
  Bed : Subsystem  mask{L=bed.floor.length, W=bed.floor.width, T_floor=bed.floor.thickness, rho_floor=bed.floor.density, color_floor=bed.floor.color, T=bed.wall.thickness, H=bed.wall.height, rho_wall=bed.wall.density, color_wall=bed.wall.color}
      mask prompts: L "Length (m)"; W "Width (m)"; T_floor "Thickness (m)"; rho_floor "Density (kg/m^3)"; color_floor "Color [R G B]"; T "Thickness (m)"; H "Height (m)"; rho_wall "Density (kg/m^3)"; color_wall "Color [R G B]"
      mask init:
      | d1 = 0.1; % width of vertical bars
      | d2 = (L - 4*d1)/3; % width of side panels
      | d3 = (W - 3*d1)/2; % width of front panels
      | d4 = T/2; % panel indentation 
      | 
      | % Wall cross-section
      | CS = zeros(40,2);
      | CS(1,:) = [L/2-T,-W/2+T];
      | CS(2,:) = [-L/2,-W/2+T];
      | CS(3,:) = [-L/2,-W/2];
      | CS(4,:) = CS(3,:) + [d1,0];
      | CS(5,:) = CS(4,:) + [0,d4];
      | CS(6,:) = CS(5,:) + [d2,0];
      | CS(7,:) = CS(6,:) + [0,-d4];
      | CS(8,:) = CS(7,:) + [d1,0];
      | CS(9,:) = CS(8,:) + [0,d4];
      | CS(10:16,:) = CS(9:-1:3,:).*[-1,1];
      | CS(17,:) = CS(16,:) + [0,d1];
      | CS(18,:) = CS(17,:) + [-d4,0];
      | CS(19,:) = CS(18,:) + [0,d3];
      | CS(20,:) = CS(19,:) + [d4,0];
      | CS(21:40,:) = CS(20:-1:1,:).*[1,-1];
      mask DialogControl Container6 Prompt: Floor
      mask DialogControl Container4 Prompt: Wall
      mask Display: image(fullfile(matlabroot,'toolbox','physmod','sm','smdemos','dump_trailer','images','sm_dump_trailer_bed.png'));
  Frame : sm_dump_trailer_lib/Frame  W=bed.frame.width  L=bed.frame.length  H=bed.frame.height  T=bed.frame.thickness  d_innerbeams=bed.frame.innerbeamdistance  rho=bed.frame.density  color=bed.frame.color
      settings: SourceProductBaseCode=MS
  Frame to Bed XForm : sm_lib/Frames and Transforms/Rigid Transform  TranslationMethod=StandardAxis  TranslationStandardOffset=bed.frame.height/2 + bed.floor.thickness/2  TranslationLengthUnit=m  TranslationStandardAxis=+Z  TranslationCartesianOffset=[0 0 0]  TranslationROffset=0  TranslationROffsetUnits=m  TranslationZOffset=0  TranslationZOffsetUnits=m  TranslationThetaOffset=0  TranslationThetaOffsetUnits=deg  RotationMethod=StandardAxis  RotationAngleUnits=deg  RotationStandardAxis=+Z  RotationAngle=-90  RotationArbitraryAxis=[0 0 1]  FollAlignAxisA=+X  BaseAlignAxisA=+Y  FollAlignAxisB=+Y  BaseAlignAxisB=+Z  RotationSequenceAxes=FollowerAxes  RotationSequence=XYX  RotationSequenceAngles=[0 0 0]  RotationSequenceAnglesUnits=deg  RotationMatrix=[1 0 0; 0 1 0; 0 0 1]
  Frame to Left Hoist XForm : sm_lib/Frames and Transforms/Rigid Transform  TranslationMethod=Cartesian  TranslationStandardOffset=0  TranslationLengthUnit=m  TranslationStandardAxis=-Z  TranslationCartesianOffset=bed.hoistbracket.offset  TranslationROffset=0  TranslationROffsetUnits=m  TranslationZOffset=0  TranslationZOffsetUnits=m  TranslationThetaOffset=0  TranslationThetaOffsetUnits=deg  RotationMethod=StandardAxis  RotationAngleUnits=deg  RotationStandardAxis=+Y  RotationAngle=180  RotationArbitraryAxis=[0 0 1]  FollAlignAxisA=+X  BaseAlignAxisA=+Y  FollAlignAxisB=+Y  BaseAlignAxisB=+Z  RotationSequenceAxes=FollowerAxes  RotationSequence=XYX  RotationSequenceAngles=[0 0 0]  RotationSequenceAnglesUnits=deg  RotationMatrix=[1 0 0; 0 1 0; 0 0 1]
  Frame to Left Rod XForm : sm_lib/Frames and Transforms/Rigid Transform  TranslationMethod=Cartesian  TranslationStandardOffset=0  TranslationLengthUnit=m  TranslationStandardAxis=-Z  TranslationCartesianOffset=bed.rodbracket.offset  TranslationROffset=0  TranslationROffsetUnits=m  TranslationZOffset=0  TranslationZOffsetUnits=m  TranslationThetaOffset=0  TranslationThetaOffsetUnits=deg  RotationMethod=StandardAxis  RotationAngleUnits=deg  RotationStandardAxis=+Y  RotationAngle=180  RotationArbitraryAxis=[0 0 1]  FollAlignAxisA=+X  BaseAlignAxisA=+Y  FollAlignAxisB=+Y  BaseAlignAxisB=+Z  RotationSequenceAxes=FollowerAxes  RotationSequence=XYX  RotationSequenceAngles=[0 0 0]  RotationSequenceAnglesUnits=deg  RotationMatrix=[1 0 0; 0 1 0; 0 0 1]
  Frame to Right Hoist XForm : sm_lib/Frames and Transforms/Rigid Transform  TranslationMethod=Cartesian  TranslationStandardOffset=0  TranslationLengthUnit=m  TranslationStandardAxis=-Z  TranslationCartesianOffset=bed.hoistbracket.offset  TranslationROffset=0  TranslationROffsetUnits=m  TranslationZOffset=0  TranslationZOffsetUnits=m  TranslationThetaOffset=0  TranslationThetaOffsetUnits=deg  RotationMethod=StandardAxis  RotationAngleUnits=deg  RotationStandardAxis=+Y  RotationAngle=180  RotationArbitraryAxis=[0 0 1]  FollAlignAxisA=+X  BaseAlignAxisA=+Y  FollAlignAxisB=+Y  BaseAlignAxisB=+Z  RotationSequenceAxes=FollowerAxes  RotationSequence=XYX  RotationSequenceAngles=[0 0 0]  RotationSequenceAnglesUnits=deg  RotationMatrix=[1 0 0; 0 1 0; 0 0 1]
  Frame to Right Rod XForm : sm_lib/Frames and Transforms/Rigid Transform  TranslationMethod=Cartesian  TranslationStandardOffset=0  TranslationLengthUnit=m  TranslationStandardAxis=-Z  TranslationCartesianOffset=bed.rodbracket.offset  TranslationROffset=0  TranslationROffsetUnits=m  TranslationZOffset=0  TranslationZOffsetUnits=m  TranslationThetaOffset=0  TranslationThetaOffsetUnits=deg  RotationMethod=StandardAxis  RotationAngleUnits=deg  RotationStandardAxis=+Y  RotationAngle=180  RotationArbitraryAxis=[0 0 1]  FollAlignAxisA=+X  BaseAlignAxisA=+Y  FollAlignAxisB=+Y  BaseAlignAxisB=+Z  RotationSequenceAxes=FollowerAxes  RotationSequence=XYX  RotationSequenceAngles=[0 0 0]  RotationSequenceAnglesUnits=deg  RotationMatrix=[1 0 0; 0 1 0; 0 0 1]
  Left Hoist Bracket : sm_dump_trailer_lib/Bracket  Hbracket=bed.hoistbracket.height  Wbracket=bed.hoistbracket.width  Tbracket=bed.hoistbracket.thickness  Hhole=bed.hoistbracket.holeheight  Rhole=bed.hoistbracket.holeradius  rho=bed.hoistbracket.density  bracketColor=bed.hoistbracket.color
      settings: SourceProductBaseCode=MS
  Left Rod Bracket : sm_dump_trailer_lib/Bracket  Hbracket=bed.rodbracket.height  Wbracket=bed.rodbracket.width  Tbracket=bed.rodbracket.thickness  Hhole=bed.rodbracket.holeheight  Rhole=bed.rodbracket.holeradius  rho=bed.rodbracket.density  bracketColor=bed.rodbracket.color
      settings: SourceProductBaseCode=MS
  Left Rod Weld : sm_lib/Joints/Weld Joint  JointMode=Normal  SenseConstraintForce=off  SenseConstraintForceX=off  SenseConstraintForceY=off  SenseConstraintForceZ=off  SenseConstraintTorque=off  SenseConstraintTorqueX=off  SenseConstraintTorqueY=off  SenseConstraintTorqueZ=off  SenseTotalForce=off  SenseTotalForceX=off  SenseTotalForceY=off  SenseTotalForceZ=off  SenseTotalTorque=off  SenseTotalTorqueX=off  SenseTotalTorqueY=off  SenseTotalTorqueZ=off  CompositeWrenchDir=FollowerOnBase  CompositeWrenchFrame=BaseFrame
  Right Hoist Bracket : sm_dump_trailer_lib/Bracket  Hbracket=bed.hoistbracket.height  Wbracket=bed.hoistbracket.width  Tbracket=bed.hoistbracket.thickness  Hhole=bed.hoistbracket.holeheight  Rhole=bed.hoistbracket.holeradius  rho=bed.hoistbracket.density  bracketColor=bed.hoistbracket.color
      settings: SourceProductBaseCode=MS
  Right Rod Bracket : sm_dump_trailer_lib/Bracket  Hbracket=bed.rodbracket.height  Wbracket=bed.rodbracket.width  Tbracket=bed.rodbracket.thickness  Hhole=bed.rodbracket.holeheight  Rhole=bed.rodbracket.holeradius  rho=bed.rodbracket.density  bracketColor=bed.rodbracket.color
      settings: SourceProductBaseCode=MS
  Right Rod Weld : sm_lib/Joints/Weld Joint  JointMode=Normal  SenseConstraintForce=off  SenseConstraintForceX=off  SenseConstraintForceY=off  SenseConstraintForceZ=off  SenseConstraintTorque=off  SenseConstraintTorqueX=off  SenseConstraintTorqueY=off  SenseConstraintTorqueZ=off  SenseTotalForce=off  SenseTotalForceX=off  SenseTotalForceY=off  SenseTotalForceZ=off  SenseTotalTorque=off  SenseTotalTorqueX=off  SenseTotalTorqueY=off  SenseTotalTorqueZ=off  CompositeWrenchDir=FollowerOnBase  CompositeWrenchFrame=BaseFrame
  Rod : Subsystem  mask{L=bed.rod.length, r=bed.rod.radius, d_bracket=bed.rod.d_bracket, d_rev=bed.rod.d_rev, rho=bed.rod.density, color=bed.rod.color}
      mask prompts: L "Length (m)"; r "Radius (m)"; d_bracket "Distance from center to bracket holes (m)"; d_rev "Distance from center to revolute joints (m)"; rho "Density (kg/m^3)"; color "Color [R G B]"
      mask Display: image(fullfile(matlabroot,'toolbox','physmod','sm','smdemos','dump_trailer','images','sm_dump_trailer_rod.png'));
  Left Rod : PMIOPort  Side=Left
  Left Hoist Hole : PMIOPort  Port=2  Side=Left
  Right Rod : PMIOPort  Port=3  Side=Right
  Right Hoist Hole : PMIOPort  Port=4  Side=Right
  connections:
  Frame to Left Rod XForm/LConn1 -- Frame/LConn3
  Left Hoist Hole/RConn1 -- Left Hoist Bracket/RConn1
  Right Hoist Bracket/RConn1 -- Right Hoist Hole/RConn1
  Frame to Right Hoist XForm/RConn1 -- Right Hoist Bracket/LConn1
  Frame to Left Hoist XForm/LConn1 -- Frame/LConn2
  Frame to Left Hoist XForm/RConn1 -- Left Hoist Bracket/LConn1
  Frame to Left Rod XForm/RConn1 -- Left Rod Bracket/LConn1
  Frame to Right Rod XForm/RConn1 -- Right Rod Bracket/LConn1
  Frame to Right Rod XForm/LConn1 -- Frame/RConn2
  Left Rod/RConn1 -- Rod/LConn2
  Right Rod Bracket/RConn1 -- Right Rod Weld/RConn1
  Right Rod/RConn1 -- Rod/RConn2
  Frame to Right Hoist XForm/LConn1 -- Frame/RConn1
  Frame to Bed XForm/LConn1 -- Frame/LConn1
  Frame to Bed XForm/RConn1 -- Bed/RConn1
  Left Rod Bracket/RConn1 -- Left Rod Weld/RConn1
  Rod/LConn1 -- Left Rod Weld/LConn1
  Right Rod Weld/LConn1 -- Rod/RConn1
